simulink model "Pulse_Cases"  (R2024b)
settings: Solver=VariableStepAuto  StartTime=0.0  StopTime=10.0  RelTol=1e-3
settings Model: Creator=HP  LastModifiedBy=HP

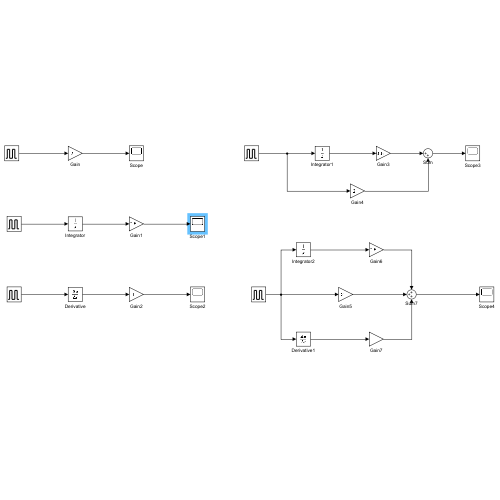
[thumbnail: Simulink's stored preview of the top-level diagram]
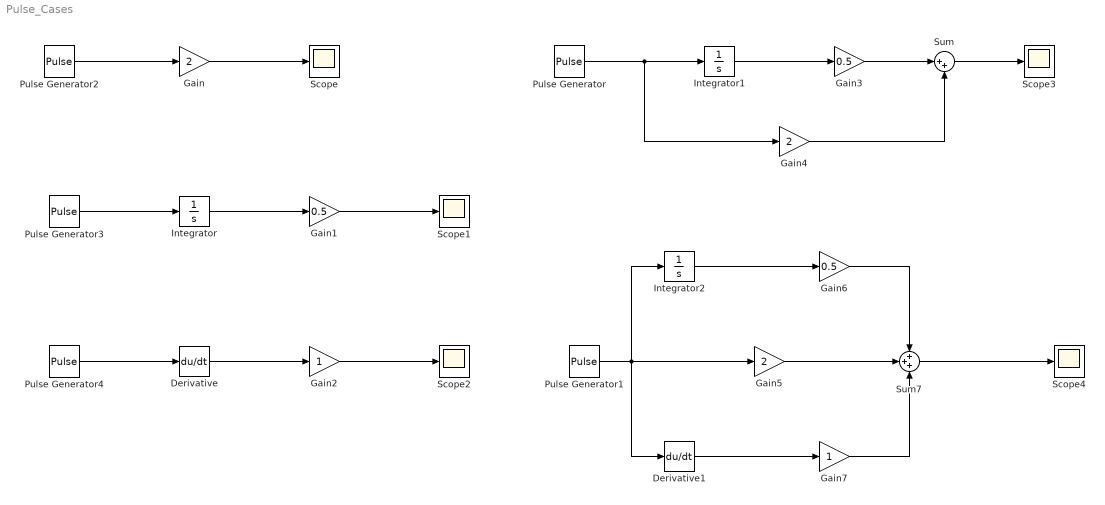
== system Pulse_Cases ==
  Derivative : Derivative
  Derivative1 : Derivative
  Gain : Gain  Gain=2
  Gain1 : Gain  Gain=0.5
  Gain2 : Gain
  Gain3 : Gain  Gain=0.5
  Gain4 : Gain  Gain=2
  Gain5 : Gain  Gain=2
  Gain6 : Gain  Gain=0.5
  Gain7 : Gain
  Integrator : Integrator
  Integrator1 : Integrator
  Integrator2 : Integrator
  Pulse Generator{,1..4} (5 alike) : DiscretePulseGenerator  PulseType=Time based  Amplitude=5  Period=10  PulseWidth=5
  Scope{,1..4} (5 alike) : Scope
  Sum : Sum  Inputs=|++
  Sum7 : Sum  Inputs=+++
  wires:
  Pulse Generator3/1 -> Integrator/1
  Pulse Generator2/1 -> Gain/1
  Pulse Generator1/1 -> Derivative1/1, Integrator2/1, Gain5/1
  Gain7/1 -> Sum7/3
  Gain2/1 -> Scope2/1
  Derivative/1 -> Gain2/1
  Sum7/1 -> Scope4/1
  Pulse Generator/1 -> Integrator1/1, Gain4/1
  Gain/1 -> Scope/1
  Gain1/1 -> Scope1/1
  Gain4/1 -> Sum/2
  Gain3/1 -> Sum/1
  Gain6/1 -> Sum7/1
  Gain5/1 -> Sum7/2
  Integrator1/1 -> Gain3/1
  Pulse Generator4/1 -> Derivative/1
  Integrator2/1 -> Gain6/1
  Sum/1 -> Scope3/1
  Integrator/1 -> Gain1/1
  Derivative1/1 -> Gain7/1
